simulink model "BallPosController"  (R2020a)
settings: Solver=VariableStepAuto  StartTime=0.0  StopTime=inf  RelTol=1e-3
settings Model: Creator=tebyb  LastModifiedBy=tebyb
settings DataIOCC: ExternalInput=XCoord, YCoord  SaveFormat=Array  SignalLogging=off  DSMLogging=off  SaveTime=off  ReturnWorkspaceOutputs=off

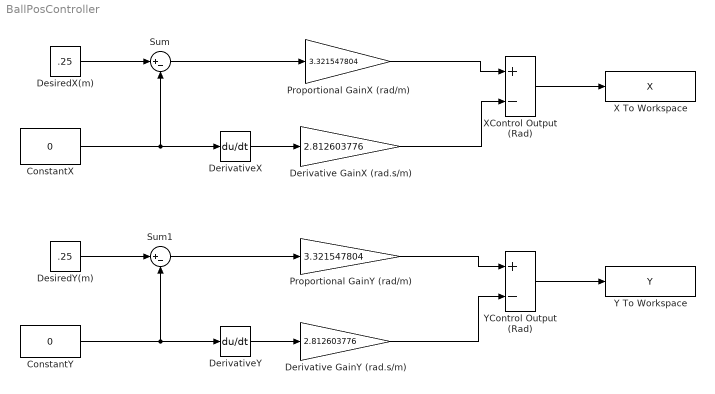
== system BallPosController ==
  ConstantX : Constant  Value=0
  ConstantY : Constant  Value=0
  Derivative GainX (rad.s/m) : Gain  Gain=2.812603776
  Derivative GainY (rad.s/m) : Gain  Gain=2.812603776
  DerivativeX : Derivative  CoefficientInTFapproximation=0
  DerivativeY : Derivative  CoefficientInTFapproximation=0
  DesiredX(m) : Constant  Value=.25
  DesiredY(m) : Constant  Value=.25
  Proportional GainX (rad/m) : Gain  Gain=3.321547804
  Proportional GainY (rad/m) : Gain  Gain=3.321547804
  Sum : Sum  Inputs=|+-
  Sum1 : Sum  Inputs=|+-
  X To Workspace : ToWorkspace  VariableName=X  SaveFormat=Timeseries  SampleTime=-1
  XControl Output (Rad) : Sum  Inputs=+-
  Y To Workspace : ToWorkspace  VariableName=Y  SaveFormat=Timeseries  SampleTime=-1
      settings: MaxDataPoints=1
  YControl Output (Rad) : Sum  Inputs=+-
  wires:
  Sum/1 -> Proportional GainX (rad/m)/1
  ConstantX/1 -> Sum/2, DerivativeX/1
  Derivative GainX (rad.s/m)/1 -> XControl Output (Rad)/2
  DesiredX(m)/1 -> Sum/1
  Proportional GainX (rad/m)/1 -> XControl Output (Rad)/1
  Proportional GainY (rad/m)/1 -> YControl Output (Rad)/1
  DesiredY(m)/1 -> Sum1/1
  Derivative GainY (rad.s/m)/1 -> YControl Output (Rad)/2
  Sum1/1 -> Proportional GainY (rad/m)/1
  ConstantY/1 -> Sum1/2, DerivativeY/1
  XControl Output (Rad)/1 -> X To Workspace/1
  YControl Output (Rad)/1 -> Y To Workspace/1
  DerivativeX/1 -> Derivative GainX (rad.s/m)/1
  DerivativeY/1 -> Derivative GainY (rad.s/m)/1
